simulink library "alfa_wall_out"  (R2013b)
settings: Solver=ode45  StartTime=0.0  StopTime=10.0  RelTol=1e-3
libraries: carnot x1
settings Model: Creator=lena.frank  LastModifiedBy=drhf

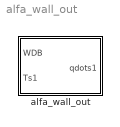
== system alfa_wall_out ==
  alfa_wall_out : Subsystem  mask(ALFA){pos=0, absorption_out=0.4, emission_out=0.7, wallsurface=1}
      mask prompts: pos "Azimut (south = 0, east = -90) in degrees"; absorption_out "Solar absorption outside (0..1)"; emission_out "Longwave emissivity of surface (0..1)"; wallsurface "Wall surface in m²"
      mask help:
      | Convective and radiative HEAT TRANSFER at the WEATHER EXPOSED SURFACE of an OUTER WALL.
      |
      | [W*] : modified weather data, adapted to height over ground,
      | Ts : temperature of outdoor wall surface, °C,
      | qdots : specific heat flow into wall / window construction, W/m^2.
      mask init:
      | if length(pos) == 1
      |     pos = [90  pos 0]; % pos is [inclination azimut rotation]
      | end

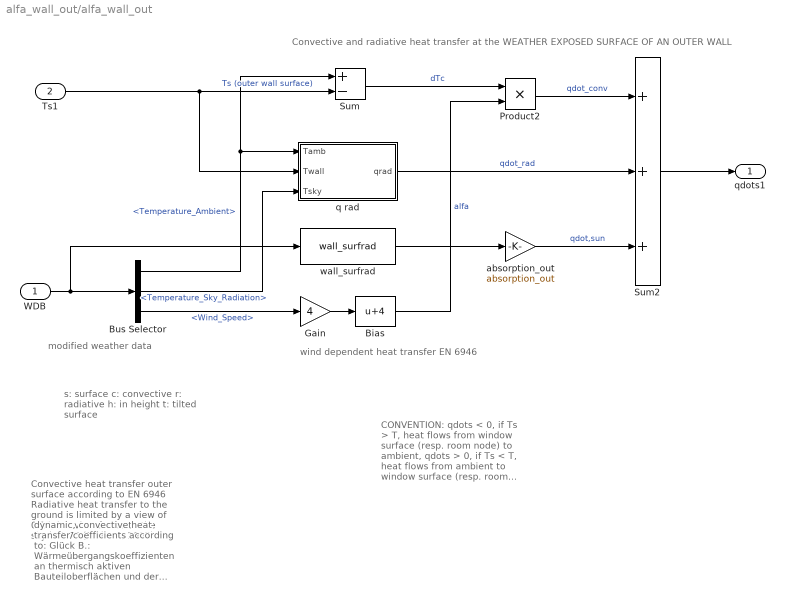
== system alfa_wall_out/alfa_wall_out ==
  note: wind dependent heat transfer EN 6946
  note: CONVENTION:
      | qdots < 0, if Ts > T, heat flows from window surface (resp. room node) to ambient,
      | qdots > 0, if Ts < T, heat flows from ambient to window surface (resp. room node).
  note: modified
      | weather data
  note: s: surface
      | c: convective
      | r: radiative
      | h: in height
      | t: tilted surface
  note: Convective and radiative heat transfer at the WEATHER EXPOSED SURFACE OF AN OUTER WALL
  note: Convective heat transfer outer surface according to EN 6946
      | Radiative heat transfer to the ground is limited by a view of 0.25, i.e. view factor to the sky is 0.75 (Frohner, 2005)
  note: dynamic, convective heat transfer coefficients according to: Glück B.: Wärmeübergangskoeffizienten an thermisch aktiven Bauteiloberflächen
      | und der Übergang zu Basiskennlinien für die Wärmestromdichte; gi Gesundheits-Ingenieur; 128. Jahrgang 2007, Heft 1, Seiten 1-10
  WDB : Inport
  Ts1 : Inport  Port=2
  Bias : Bias  Bias=4
  Bus Selector : BusSelector  OutputSignals=Temperature_Ambient,Temperature_Sky_Radiation,Wind_Speed
  Gain : Gain  Gain=4
  Product2 : Product  SaturateOnIntegerOverflow=on  RndMeth=Zero  InputSameDT=on  OutDataTypeStr=Inherit: Same as first input
  Sum : Sum  Inputs=+-  SaturateOnIntegerOverflow=on  InputSameDT=on  OutDataTypeStr=Inherit: Same as first input
  Sum2 : Sum  Inputs=+++  SaturateOnIntegerOverflow=on  InputSameDT=on  OutDataTypeStr=Inherit: Same as first input
  absorption_out : Gain  Gain=absorption_out  SaturateOnIntegerOverflow=on  OutDataTypeStr=Inherit: Same as input  ParamDataTypeStr=Inherit: Same as input
  q rad : Subsystem
  wall_surfrad : carnot/Load/Houses/heat_transfer/wall_surfrad  pos=pos
  qdots1 : Outport
  wires:
  q rad/1(qrad) -> Sum2/2  "qdot_rad"
  Product2/1 -> Sum2/1  "qdot_conv"
  absorption_out/1 -> Sum2/3  "qdot,sun"
  Bias/1 -> Product2/2  "alfa"
  wall_surfrad/1 -> absorption_out/1
  Ts1/1 -> q rad/2(Twall), Sum/2  "Ts (outer wall surface)"
  Sum2/1 -> qdots1/1
  WDB/1 -> Bus Selector/1, wall_surfrad/1
  Sum/1 -> Product2/1  "dTc"
  Bus Selector/1 -> Sum/1, q rad/1(Tamb)  "<Temperature_Ambient>"
  Bus Selector/2 -> q rad/3(Tsky)  "<Temperature_Sky_Radiation>"
  Bus Selector/3 -> Gain/1  "<Wind_Speed>"
  Gain/1 -> Bias/1

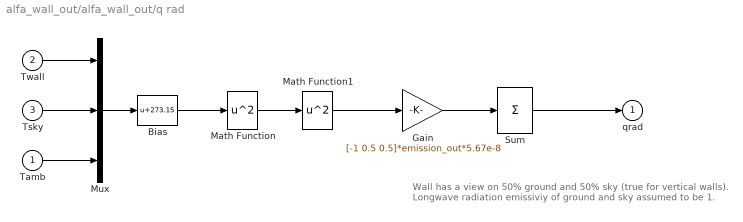
== system alfa_wall_out/alfa_wall_out/q rad ==
  note: Wall has a view on 50% ground and 50% sky (true for vertical walls).
      | Longwave radiation emissiviy of ground and sky assumed to be 1.
  Tamb : Inport
  Twall : Inport  Port=2
  Tsky : Inport  Port=3
  Bias : Bias  Bias=273.15
  Gain : Gain  Gain=[-1 0.5 0.5]*emission_out*5.67e-8
  Math Function : Math  Operator=square  SaturateOnIntegerOverflow=on
  Math Function1 : Math  Operator=square  SaturateOnIntegerOverflow=on
  Mux : Mux  Inputs=3
  Sum : Sum  Inputs=1  SaturateOnIntegerOverflow=on  InputSameDT=on  OutDataTypeStr=Inherit: Same as first input
  qrad : Outport
  wires:
  Tsky/1 -> Mux/2
  Tamb/1 -> Mux/3
  Sum/1 -> qrad/1
  Twall/1 -> Mux/1
  Bias/1 -> Math Function/1
  Mux/1 -> Bias/1
  Math Function/1 -> Math Function1/1
  Gain/1 -> Sum/1
  Math Function1/1 -> Gain/1
